simulink model "biped_sim"  (R2016a)
settings: Solver=FixedStepAuto  StartTime=0.0  StopTime=inf  FixedStep=Ts/16  MaxStep=Ts  MinStep=Ts/4  RelTol=1e-3
PreLoadFcn:
  | clear
  | biped_setup
values from neighbouring files (symbols this model uses):
  a = 2*pi*freq*obj.Ts/(2*pi*freq*obj.Ts + 1)    [StateEstimator.m]
  env = struct()    [BipedController.m]    (also in biped_setup.m = Environment())
  ground_data = zeros(2, 5)    [BipedVisualization.m]    (also in Planner.m; biped_setup.m = [ground_x, ground_y, ground_stiffness, ground_damping, groun)
  Ts = 1e-3    (= 0.001)    [BipedController.m]    (also in Planner.m = 0.1; Sequencing.m; StateEstimator.m)
  X0 = struct()    [RobotState.m]    (also in biped_setup.m = RobotState())
settings Model: Creator=patrick  LastModifiedBy=robot
settings SolverCC: InitialStep=Ts  InsertRTBMode=Always
settings DataIOCC: SaveOutput=off  SaveTime=off
settings DebuggingCC: ReadBeforeWriteMsg=DisableAll  WriteAfterWriteMsg=DisableAll  WriteAfterReadMsg=DisableAll  MultiTaskDSMMsg=none  UnnecessaryDatatypeConvMsg=warning  VectorMatrixConversionMsg=warning  BusObjectLabelMismatch=none  AllowSymbolicDim=off
settings ModelReferenceCC: UpdateModelReferenceTargets=IfOutOfDate  PropagateSignalLabelsOutOfModel=off
settings SFSimCC: SFSimEcho=off
settings GRTTargetCC: GeneratePreprocessorConditionals=Use local settings

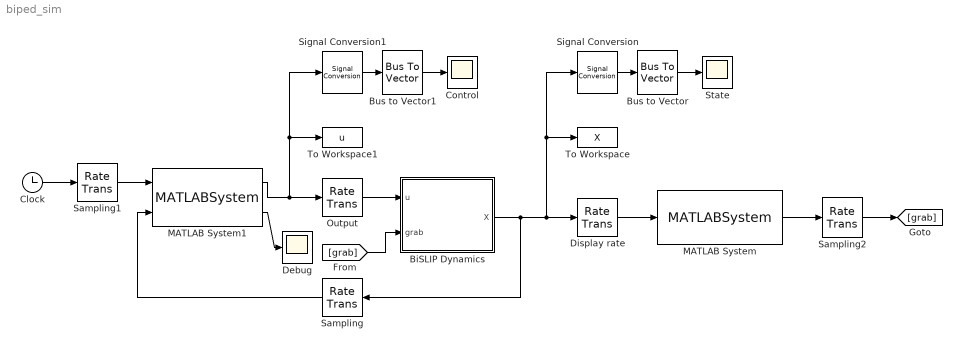
== system biped_sim ==
  BiSLIP Dynamics : Subsystem
  Bus to Vector : BusToVector
  Bus to Vector1 : BusToVector
  Clock : Clock
  Control : Scope
  Debug : Scope
  Display rate : RateTransition  X0=X0  OutPortSampleTime=Ts*16
  MATLAB System : MATLABSystem  System=BipedVisualization  env=env  ground_data=ground_data  SimulateUsing=Interpreted execution
      mask Type: BipedVisualization
      mask Display:
      | disp('BipedVisualization');
      | port_label('input',1,'X');
      | port_label('output',1,'v');
  MATLAB System1 : MATLABSystem  System=BipedController  Ts=Ts  env=env  phase_rate=2  target_dx=1  SimulateUsing=Code generation
      mask Type: BipedController
      mask Display:
      | disp('BipedController');
      | port_label('input',1,'t');
      | port_label('input',2,'X');
      | port_label('output',1,'u');
      | port_label('output',2,'dbg');
  Output : RateTransition  OutPortSampleTimeOpt=Inherit  OutPortSampleTime=-a
  Sampling : RateTransition  OutPortSampleTime=Ts
  Sampling1 : RateTransition  OutPortSampleTime=Ts
  Sampling2 : RateTransition  OutPortSampleTimeOpt=Inherit  OutPortSampleTime=Ts/16
  Signal Conversion : SignalConversion  ConversionOutput=Virtual bus  OverrideOpt=off
  Signal Conversion1 : SignalConversion  ConversionOutput=Virtual bus  OverrideOpt=off
  State : Scope
  To Workspace : ToWorkspace  VariableName=X  SaveFormat=Timeseries  SampleTime=-1
      settings: MaxDataPoints=1e6
  To Workspace1 : ToWorkspace  VariableName=u  SaveFormat=Timeseries  SampleTime=-1
      settings: MaxDataPoints=1e6
  wires:
  Output/1 -> BiSLIP Dynamics/1(u)
  MATLAB System1/1 -> Signal Conversion1/1, To Workspace1/1, Output/1
  BiSLIP Dynamics/1(X) -> Signal Conversion/1, To Workspace/1, Display rate/1, Sampling/1
  Sampling/1 -> MATLAB System1/2
  Clock/1 -> Sampling1/1
  Sampling1/1 -> MATLAB System1/1
  [grab] -> BiSLIP Dynamics/2(grab)
  Signal Conversion/1 -> Bus to Vector/1
  Bus to Vector/1 -> State/1
  Signal Conversion1/1 -> Bus to Vector1/1
  Bus to Vector1/1 -> Control/1
  MATLAB System/1 -> Sampling2/1
  Display rate/1 -> MATLAB System/1
  Sampling2/1 -> [grab]
  MATLAB System1/2 -> Debug/1

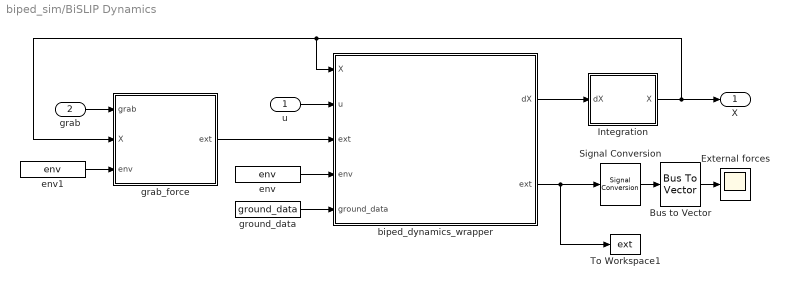
== system biped_sim/BiSLIP Dynamics ==
  u : Inport
  grab : Inport  Port=2
  Bus to Vector : BusToVector
  External forces : Scope
  Integration : Subsystem
  Signal Conversion : SignalConversion  ConversionOutput=Virtual bus  OverrideOpt=off
  To Workspace1 : ToWorkspace  VariableName=ext  SaveFormat=Timeseries  SampleTime=-1
      settings: MaxDataPoints=1e6
  biped_dynamics_wrapper : MATLAB Function  TreatAsAtomicUnit=on
      settings: PermitHierarchicalResolution=ParametersOnly
  env : Constant  Value=env  OutDataTypeStr=Bus: environment_bus
  env1 : Constant  Value=env  OutDataTypeStr=Bus: environment_bus
  grab_force : MATLAB Function  TreatAsAtomicUnit=on
      settings: PermitHierarchicalResolution=ParametersOnly
  ground_data : Constant  Value=ground_data
  X : Outport
  wires:
  u/1 -> biped_dynamics_wrapper/2(u)
  env/1 -> biped_dynamics_wrapper/4(env)
  ground_data/1 -> biped_dynamics_wrapper/5(ground_data)
  grab/1 -> grab_force/1(grab)
  grab_force/1(ext) -> biped_dynamics_wrapper/3("ext ")
  env1/1 -> grab_force/3(env)
  Integration/1(X) -> X/1, grab_force/2(X), biped_dynamics_wrapper/1(X)
  biped_dynamics_wrapper/1(dX) -> Integration/1(dX)
  Signal Conversion/1 -> Bus to Vector/1
  biped_dynamics_wrapper/2(ext) -> To Workspace1/1, Signal Conversion/1
  Bus to Vector/1 -> External forces/1

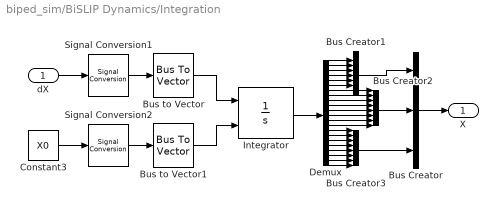
== system biped_sim/BiSLIP Dynamics/Integration ==
  dX : Inport
  Bus Creator : BusCreator  Inputs=3  OutDataTypeStr=Bus: state_bus  NonVirtualBus=on
  Bus Creator1 : BusCreator  Inputs=6  OutDataTypeStr=Bus: body  NonVirtualBus=on
  Bus Creator2 : BusCreator  Inputs=8  OutDataTypeStr=Bus: right  NonVirtualBus=on
  Bus Creator3 : BusCreator  Inputs=8  OutDataTypeStr=Bus: left  NonVirtualBus=on
  Bus to Vector : BusToVector
  Bus to Vector1 : BusToVector
  Constant3 : Constant  Value=X0  OutDataTypeStr=Bus: state_bus
  Demux : Demux  Outputs=22
  Integrator : Integrator  InitialConditionSource=external  InitialCondition=X0
  Signal Conversion1 : SignalConversion  ConversionOutput=Virtual bus  OverrideOpt=off
  Signal Conversion2 : SignalConversion  ConversionOutput=Virtual bus  OverrideOpt=off
  X : Outport
  wires:
  Bus to Vector/1 -> Integrator/1
  Bus to Vector1/1 -> Integrator/2
  Constant3/1 -> Signal Conversion2/1
  Signal Conversion1/1 -> Bus to Vector/1
  Signal Conversion2/1 -> Bus to Vector1/1
  dX/1 -> Signal Conversion1/1
  Integrator/1 -> Demux/1
  Bus Creator/1 -> X/1
  Demux/1 -> Bus Creator1/1
  Demux/2 -> Bus Creator1/2
  Demux/3 -> Bus Creator1/3
  Demux/4 -> Bus Creator1/4
  Demux/5 -> Bus Creator1/5
  Demux/6 -> Bus Creator1/6
  Demux/7 -> Bus Creator2/1
  Demux/8 -> Bus Creator2/2
  Demux/9 -> Bus Creator2/3
  Demux/10 -> Bus Creator2/4
  Demux/11 -> Bus Creator2/5
  Demux/12 -> Bus Creator2/6
  Demux/13 -> Bus Creator2/7
  Demux/14 -> Bus Creator2/8
  Demux/15 -> Bus Creator3/1
  Demux/16 -> Bus Creator3/2
  Demux/17 -> Bus Creator3/3
  Demux/18 -> Bus Creator3/4
  Demux/19 -> Bus Creator3/5
  Demux/20 -> Bus Creator3/6
  Demux/21 -> Bus Creator3/7
  Demux/22 -> Bus Creator3/8
  Bus Creator3/1 -> Bus Creator/3
  Bus Creator2/1 -> Bus Creator/2
  Bus Creator1/1 -> Bus Creator/1

== matlab function biped_sim/BiSLIP Dynamics/biped_dynamics_wrapper ==
  data: X input Bus: state_bus; u input Bus: control_bus; dX output Bus: state_bus; ext input Bus: external_force_bus; env input Bus: environment_bus; ground_data input; ext output
function [dX, ext] = biped_dynamics_wrapper(X, u, ext, env, ground_data) %#codegen

[dX, ext] = biped_dynamics(X, u, ext, env, ground_data);

== matlab function biped_sim/BiSLIP Dynamics/grab_force ==
  data: grab input; ext output Bus: external_force_bus; X input Bus: state_bus; env input Bus: environment_bus
function ext = grab_force(grab, X, env) %#codegen

kp_f_ext = 1e4;
kd_f_ext = 2*sqrt(kp_f_ext*env.body.mass);
 
ext.body.x     = 0;
ext.body.y     = 0;
ext.body.theta = 0;
ext.right.x    = 0;
ext.right.y    = 0;
ext.left.x     = 0;
ext.left.y     = 0;

if any(grab ~= 0)
    ext.body.x = (kp_f_ext * grab(1)) - (kd_f_ext * X.body.dx);
    ext.body.y = (kp_f_ext * grab(2)) - (kd_f_ext * X.body.dy);
end
